simulink model "Cholesky_Ex4"  (R2025a)
settings: Solver=VariableStepAuto  StartTime=0.0  StopTime=10  RelTol=1e-3
InitFcn:
  | A = single(rand(16,16));
undefined symbols (not defined in the file): S, static_input_Convolution_Stream_Ex1, Subsystem, vsva2197, xcvc1902
libraries: aieUtilities x3, aieSolver x1, vmcUtilities x1
settings Model: Creator=sdegala  LastModifiedBy=sdegala
settings ModelReferenceCC: EnableRefExpFcnMdlSchedulingChecks=on
settings RTWCC: GPUComputeCapability=3.5

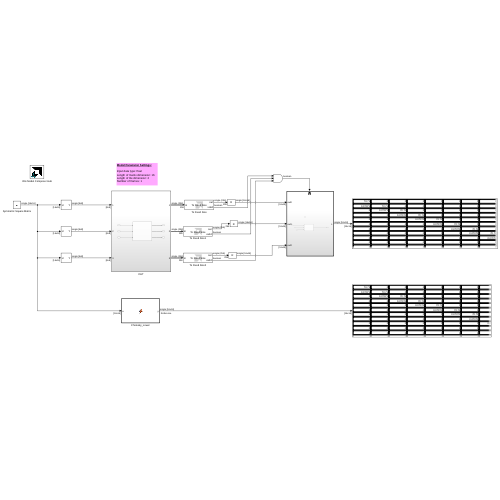
[thumbnail: Simulink's stored preview of the top-level diagram]
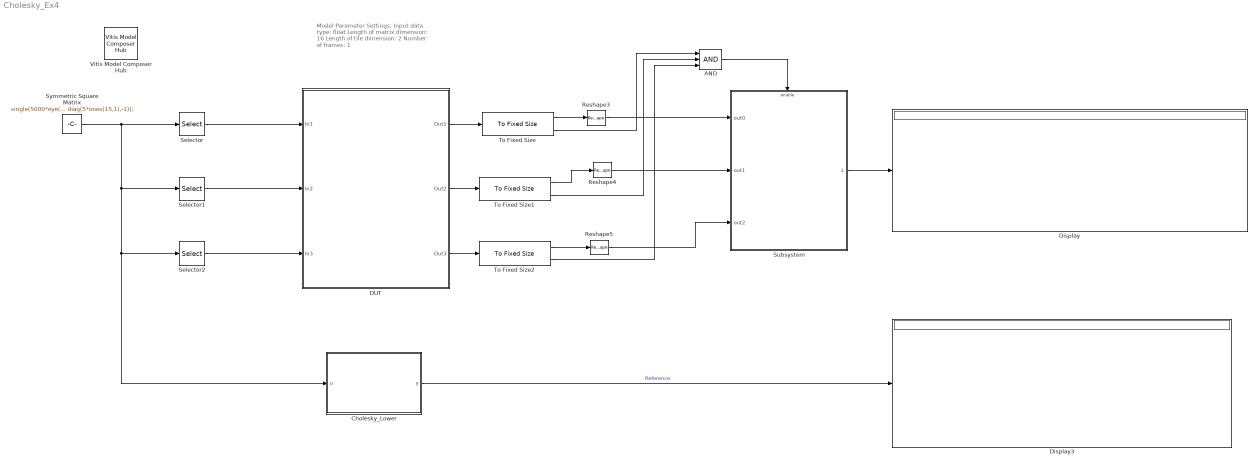
== system Cholesky_Ex4 ==
  note: Model Parameter Settings:
      |
      | Input data type: float
      | Length of matrix dimension: 16
      | Length of tile dimension: 2
      | Number of frames: 1
  AND : Logic  Inputs=3  IconShape=distinctive  AllPortsSameDT=off  OutDataTypeStr=boolean
  Cholesky_Lower : MATLAB Function  TreatAsAtomicUnit=on
  DUT : Subsystem
  Display : Display
  Display3 : Display
  Reshape3 : Reshape  OutputDimensionality=Customize  OutputDimensions=[16,16]
  Reshape4 : Reshape  OutputDimensionality=Customize  OutputDimensions=[16,16]
  Reshape5 : Reshape  OutputDimensionality=Customize  OutputDimensions=[16,16]
  Selector : Selector  NumberOfDimensions=2  InputPortWidth=3  IndexOptions=Index vector (dialog),Index vector (dialog)  Indices=1:1:8,1:1:8  OutputSizes=1,1
  Selector1 : Selector  NumberOfDimensions=2  InputPortWidth=3  IndexOptions=Index vector (dialog),Index vector (dialog)  Indices=9:1:16,1:1:8  OutputSizes=1,1
  Selector2 : Selector  NumberOfDimensions=2  InputPortWidth=3  IndexOptions=Index vector (dialog),Index vector (dialog)  Indices=9:1:16,9:1:16  OutputSizes=1,1
  Subsystem : Subsystem
  Symmetric Square Matrix : Constant  Value=single(5000*eye(16) + diag(5*ones(15,1),1) + diag(5*ones(15,1),-1));  OutDataTypeStr=single  SampleTime=1
  To Fixed Size : aieUtilities/To Fixed Size  Mode=Produce a valid output signal  OutputSize=Inherit: Same as input  CopyMethod=Buffer samples to form output  HasStatusOutput=on
  To Fixed Size1 : aieUtilities/To Fixed Size  Mode=Produce a valid output signal  OutputSize=Inherit: Same as input  CopyMethod=Buffer samples to form output  HasStatusOutput=on
  To Fixed Size2 : aieUtilities/To Fixed Size  Mode=Produce a valid output signal  OutputSize=Inherit: Same as input  CopyMethod=Buffer samples to form output  HasStatusOutput=on
  Vitis Model Composer Hub : vmcUtilities/Vitis Model Composer Hub  Tag=genX  CodeGeneration=off  SubsystemName=Subsystem  BlockHierPath=static_input_Convolution_Stream_Ex1/Subsystem  SubsystemType=AIENode  AIEArrayConfig=Use entire AIE array  StartColumn=1  NumberOfColumns=1  TargetDirectory=./code  exportDesign=on  analyzeDesign=off  validateDesignOnHw=off  ExportType=AI Engines  IpVendor=xilinx.com  IpLibrary=hls  IpVersion=1.0  IpHWLanguage=Verilog  AieCompilerOptions={}  AieSimulatorOptions={}  CreateTestbench=on  TestbenchStackSize=10  RunRtlSim=off  RunCSim=off  RunAieSim=off  enableSimulationTimeout=on  enableGraphIterations=on  AieSimTimeout=50000  AieGraphIterations=-1  RunAieSimProfiling=off  LaunchVitisAnalyzer=off  PlotOutput=off  RunX86Sim=off  X86SimTimeout=10  GenHwImage=off  GenLibadfXo=off  GenHwValidationCode=off  PlatformType=Not Specified  HwSystemType=Baremetal  HwValidationTarget=hw  ProjDevice=xcvc1902-vsva2197-1LP-e-S  ProjDevicePart=xcvc1902-vsva2197-1LP-e-S  AIEType=AIE  SamplePeriod=-1  ClockFrequency=200  DataPathParallelism=1  xilinxfamily=versalaicore  part=xcvc1902  speed=-1LP-e-S  package=vsva2197  directory=./netlist  testbench=off  incr_netlist=off  synthesis_tool=Vivado  clock_wrapper=Clock Enables  dbl_ovrd=According to Block Masks  dcm_input_clock_period=10  sysclk_period=10  simulink_period=1  eval_field=0  IPInfoJsonString="{\"DUTSubsystemName\":\"Subsystem\",\"AIESubsystem\":{\"SubsystemName\":\"Subsystem\",\"TargetDirectory\":\"./code\",\"AIEArrayConfig\":\"Use entire AIE array\",\"StartColumn\":\"0\",\"NumberOfColumns\":\"1\"},\"SubsystemTag\":\"AIENode\"}"  LogFileName=/tmp/CR-1250814/code/model_composer.log  NThreads=4  IPConfigFile=/tmp/vmctmp-13380004059271250980/static_input_Convolution_Stream_Ex1_ipconfig.json
  wires:
  DUT/1(Out1) -> To Fixed Size/1
  Symmetric Square Matrix/1 -> Selector/1, Selector1/1, Selector2/1, Cholesky_Lower/1(u)
  DUT/3(Out3) -> To Fixed Size2/1
  DUT/2(Out2) -> To Fixed Size1/1
  Cholesky_Lower/1(y) -> Display3/1  "Reference"
  Reshape3/1 -> Subsystem/1(out0)
  Reshape4/1 -> Subsystem/2(out1)
  Reshape5/1 -> Subsystem/3(out2)
  Subsystem/1(L) -> Display/1
  To Fixed Size/2 -> AND/1
  To Fixed Size1/2 -> AND/2
  To Fixed Size2/2 -> AND/3
  AND/1 -> Subsystem/Enable
  Selector/1 -> DUT/1(In1)
  Selector1/1 -> DUT/2(In2)
  Selector2/1 -> DUT/3(In3)
  To Fixed Size/1 -> Reshape3/1
  To Fixed Size1/1 -> Reshape4/1
  To Fixed Size2/1 -> Reshape5/1

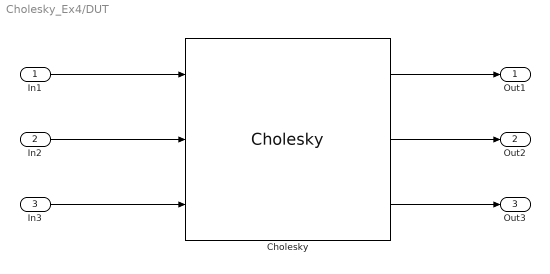
== system Cholesky_Ex4/DUT ==
  In1 : Inport
  In2 : Inport  Port=2
  In3 : Inport  Port=3
  Cholesky : aieSolver/Cholesky  AIE_VARIANT=1  data_type=float  dim_matrix=16  grid_dimension=2  num_frames=1  casc_length=1  inversion_diag=off  blockJsonConstraints=[]  blockJsonConstraintsInternal=[]  spec=vmc_cholesky.json  SerializedMaskParamNames=[]  SerializedMaskParamValues=[]  SerializedMaskParamVisibilities=[]  block_type=Cholesky  SerializedMaskParamDataypes=uint|typename|uint|uint|uint|uint|uint  SerializedMaskParamEnumStrArr=0|0|0|0|0|0|0  SerializedMaskParamEnumValArr=0|0|0|0|0|0|0  SerializedMaskParamVectorArr=0|0|0|0|0|0|0  SerializedMaskParamKeys=AIE_VARIANT|TT_DATA|TP_DIM|TP_GRID_DIM|TP_NUM_FRAMES|TP_CASC_LEN|TP_DIAG_INV
  Out1 : Outport
  Out2 : Outport  Port=2
  Out3 : Outport  Port=3
  wires:
  Cholesky/1 -> Out1/1
  In1/1 -> Cholesky/1
  In2/1 -> Cholesky/2
  In3/1 -> Cholesky/3
  Cholesky/2 -> Out2/1
  Cholesky/3 -> Out3/1

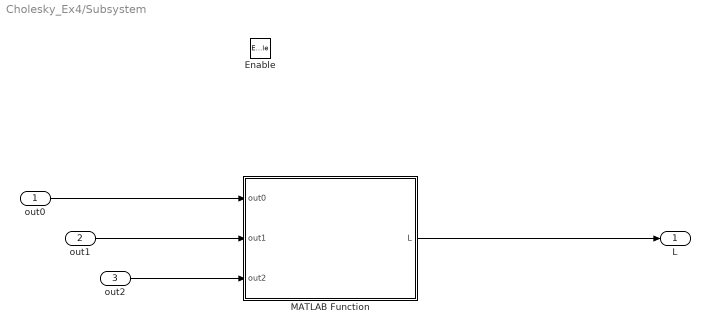
== system Cholesky_Ex4/Subsystem ==
  out0 : Inport
  out1 : Inport  Port=2
  out2 : Inport  Port=3
  Enable : EnablePort
  MATLAB Function : MATLAB Function  TreatAsAtomicUnit=on
  L : Outport
  wires:
  out0/1 -> MATLAB Function/1(out0)
  out2/1 -> MATLAB Function/3(out2)
  out1/1 -> MATLAB Function/2(out1)
  MATLAB Function/1(L) -> L/1

== matlab function Cholesky_Ex4/Subsystem/MATLAB Function ==
  data: out0 input; L output; out1 input; out2 input
function L = formCholeskyOutput(out0, out1, out2)
    block0 = reshape(out0(1:64), 8, 8);
    block1 = reshape(out1(1:64), 8, 8);
    block2 = reshape(out2(1:64), 8, 8);

    L = zeros(16, 16, 'single');

    L(1:8, 1:8)     = block0;
    L(9:16, 1:8)    = block1;
    L(9:16, 9:16)   = block2;
end

== matlab function Cholesky_Ex4/Cholesky_Lower ==
  data: u input; y output
function y = fcn(u)

y = single(chol(u,'lower'));
